simulink model "Motor_ideal_discretizado"  (R2021a)
settings: Solver=VariableStepAuto  StartTime=0.0  StopTime=10.0  RelTol=1e-3
values from neighbouring files (symbols this model uses):
  A = [0  1; 0  -125.59]    [modelo_ideal_Practica6.mat]    (also in modelo_practica4_workspace.mat; modelo_real_practica5_workspace.mat)
  B = [0 132500]    [modelo_ideal_Practica6.mat]    (also in modelo_practica4_workspace.mat; modelo_real_practica5_workspace.mat)
  C = [1 0]    [modelo_ideal_Practica6.mat]    (also in modelo_practica4_workspace.mat; modelo_real_practica5_workspace.mat)
  K = [-3.78656830443e-05 4.70346663172e-05]    [modelo_ideal_Practica6.mat]    (also in modelo_practica4_workspace.mat = [0.0297600907547 -0.00189569811321]; modelo_real_practica5_workspace.mat)
  L = [-1.20402629539 1.69403138607]    [modelo_ideal_Practica6.mat]    (also in modelo_practica4_workspace.mat = [-251.18 35488.908225]; modelo_real_practica5_workspace.mat)
  T = 0.005    [modelo_ideal_Practica6.mat]    (also in modelo_ideal_practica3_workspace.mat = 0.001; modelo_real_practica5_workspace.mat)
  Vmax = 12    [modelo_ideal_practica3_workspace.mat]
undefined symbols (not defined in the file or in its folder): Ke, P
libraries: simulink x1
settings Model: Creator=Marcial  LastModifiedBy=Marcial

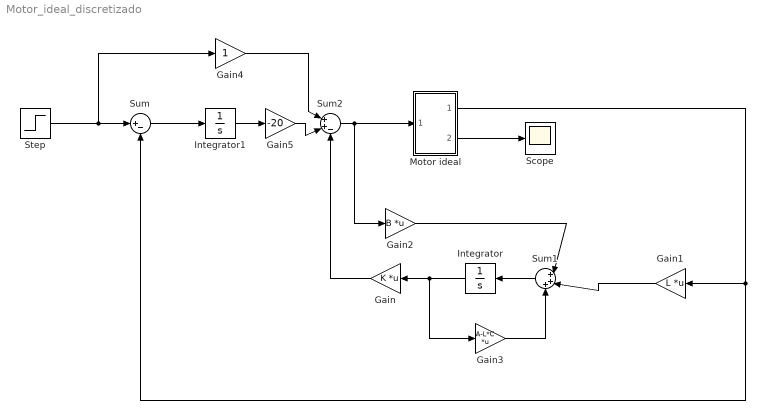
== system Motor_ideal_discretizado ==
  Gain : Gain  Gain=K  Multiplication=Matrix(K*u)
  Gain1 : Gain  Gain=L  Multiplication=Matrix(K*u)
  Gain2 : Gain  Gain=B  Multiplication=Matrix(K*u)
  Gain3 : Gain  Gain=A-L*C  Multiplication=Matrix(K*u)
  Gain4 : Gain
  Gain5 : Gain  Gain=-20
  Integrator : Integrator
  Integrator1 : Integrator
  Motor ideal : Subsystem
  Scope : Scope
  Step : Step  Time=0  SampleTime=0
  Sum : Sum  Inputs=|+-
  Sum1 : Sum  Inputs=|+++
  Sum2 : Sum  Inputs=|++-
  wires:
  ? -> ?
  Motor ideal/1(Posición) -> Gain1/1, Sum/2
  Gain/1 -> Sum2/3
  Sum/1 -> Integrator1/1
  Gain4/1 -> Sum2/1
  Integrator/1 -> Gain/1, Gain3/1
  Gain3/1 -> Sum1/3
  Step/1 -> Gain4/1, Sum/1
  Sum1/1 -> Integrator/1
  Sum2/1 -> Motor ideal/1(In1), Gain2/1
  Gain2/1 -> Sum1/1
  Gain1/1 -> Sum1/2
  Gain5/1 -> Sum2/2
  Motor ideal/2(Velocidad) -> Scope/1
  Integrator1/1 -> Gain5/1

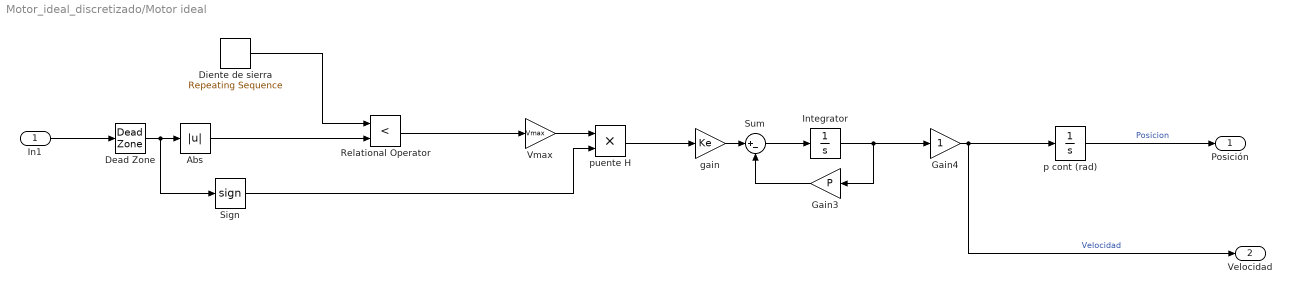
== system Motor_ideal_discretizado/Motor ideal ==
  In1 : Inport
  Abs : Abs
  Dead Zone : DeadZone  SaturateOnIntegerOverflow=on
  Diente de sierra : simulink/Sources/Repeating Sequence  rep_seq_t=linspace(0,T,100)  rep_seq_y=linspace(0,Vmax,100)
  Gain3 : Gain  Gain=P
  Gain4 : Gain
  Integrator : Integrator
  Relational Operator : RelationalOperator  Operator=<  OutDataTypeStr=boolean  RndMeth=Simplest
  Sign : Signum
  Sum : Sum  Inputs=|+-
  Vmax : Gain  Gain=Vmax
  gain : Gain  Gain=Ke
  p cont (rad) : Integrator
  puente H : Product
  Posición : Outport
  Velocidad : Outport  Port=2
  wires:
  Dead Zone/1 -> Sign/1, Abs/1
  Gain4/1 -> Velocidad/1, p cont (rad)/1  "Velocidad"
  Vmax/1 -> puente H/1
  gain/1 -> Sum/1
  Diente de sierra/1 -> Relational Operator/1
  Gain3/1 -> Sum/2
  puente H/1 -> gain/1
  Integrator/1 -> Gain3/1, Gain4/1
  Sum/1 -> Integrator/1
  Abs/1 -> Relational Operator/2
  Relational Operator/1 -> Vmax/1
  Sign/1 -> puente H/2
  In1/1 -> Dead Zone/1
  p cont (rad)/1 -> Posición/1  "Posicion"
